simulink model "PhanHoiTrangThaiGanDiemCuc2"  (R2014a)
settings: Solver=ode45  StartTime=0.0  StopTime=10.0  RelTol=1e-3
settings Model: Creator=tri  LastModifiedBy=tri

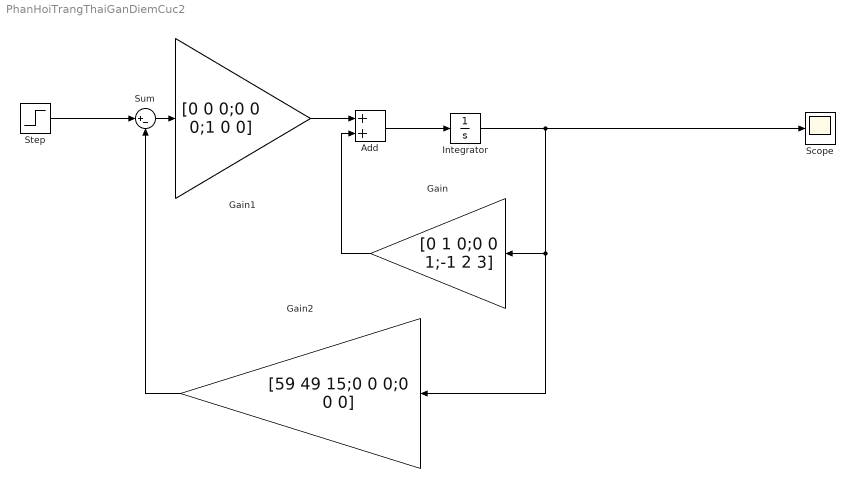
== system PhanHoiTrangThaiGanDiemCuc2 ==
  Add : Sum
  Gain : Gain  Gain=[0 1 0;0 0 1;-1 2 3]
  Gain1 : Gain  Gain=[0 0 0;0 0 0;1 0 0]
  Gain2 : Gain  Gain=[59 49 15;0 0 0;0 0 0]
  Integrator : Integrator
  Scope : Scope
  Step : Step  After=10  SampleTime=0
  Sum : Sum  Inputs=|+-
  wires:
  Gain/1 -> Add/2
  Add/1 -> Integrator/1
  Gain1/1 -> Add/1
  Integrator/1 -> Scope/1, Gain2/1, Gain/1
  Gain2/1 -> Sum/2
  Sum/1 -> Gain1/1
  Step/1 -> Sum/1
